simulink model "debounce_PP"  (R2017b)
settings: Solver=FixedStepDiscrete  StartTime=0.0  StopTime=10.0  RelTol=1e-3  EnableMultiTasking=on
model workspace (MAT data in the model file):
  already_pp = 1
Description:
  | Property Proving with an Assumption Block
  | 
  | This example shows how to perform a Simulink Design Verifier property proof using a
  | Proof Assumption block.
settings Model: Creator=The MathWorks, Inc.  LastModifiedBy=hbourbou
settings SolverCC: InsertRTBMode=Auto
settings DataIOCC: LimitDataPoints=on  SaveFormat=Structure
settings OptimizationCC: DefaultParameterBehavior=Inlined  ExpressionDepthLimit=2147483647  InitFltsAndDblsToZero=on  EfficientMapNaN2IntZero=off  LifeSpan=inf
settings DebuggingCC: AlgebraicLoopMsg=error  SaveWithParameterizedLinksMsg=none  UnderspecifiedInitializationDetection=Classic  MergeDetectMultiDrivingBlocksExec=none  SignalResolutionControl=TryResolveAllWithWarning  SolverPrmCheckMsg=warning  FcnCallInpInsideContextMsg=warning  StateNameClashWarn=warning  StrictBusMsg=Warning  SFUnexpectedBacktrackingDiag=warning  SFNoUnconditionalDefaultTransitionDiag=warning  SFExecutionAtInitializationDiag=none
settings HardwareCC: ProdBitPerPointer=32  ProdBitPerSizeT=32  ProdBitPerPtrDiffT=32  ProdLargestAtomicFloat=None  ProdIntDivRoundTo=Undefined  ProdEndianess=Unspecified  ProdWordSize=32  ProdHWDeviceType=32-bit Generic
settings ModelReferenceCC: PropagateSignalLabelsOutOfModel=off
settings SFSimCC: SimParseCustomCode=off
settings CodeAppCC: StateflowObjectComments=on
settings GRTTargetCC: TargetFcnLib=ansi_tfl_tmw.mat  TargetLangStandard=C89/C90 (ANSI)  GeneratePreprocessorConditionals=Disable all  CombineOutputUpdateFcns=off  GRTInterface=on
settings ConfigComp: DVMode=PropertyProving  DVMaxProcessTime=60  DVMakeOutputFilesUnique=off  DVParameters=on  DVModelCoverageObjectives=MCDC  DVMaxTestCaseSteps=500  DVTestSuiteOptimization=CombinedObjectives  DVAssertions=EnableAll  DVProofAssumptions=EnableAll  DVDetectActiveLogic=on  DVDetectFloatOverflow=off  DVProvingStrategy=FindViolation  DVModelReferenceHarness=on

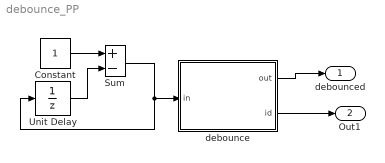
== system debounce_PP ==
  Constant : Constant  OutDataTypeStr=uint8
  Sum : Sum  Inputs=+-  OutDataTypeStr=double
  Unit Delay : UnitDelay  InitialCondition=uint8(0)  SampleTime=-1
  debounce : Stateflow chart  TreatAsAtomicUnit=on
  debounced : Outport  OutDataTypeStr=double
  Out1 : Outport  Port=2
  wires:
  Sum/1 -> Unit Delay/1, debounce/1(in)
  debounce/1(out) -> debounced/1
  debounce/2(id) -> Out1/1
  Unit Delay/1 -> Sum/2
  Constant/1 -> Sum/1

== stateflow chart debounce_PP/debounce ==
  settings: updateMethod=DISCRETE
  state To
    state To_on
      en: id = 2;
      exit: id = 0;
    state To_off
      en: id = 3;
      exit: id = 0;
  state Off
    en: out = 0 ;
    id = 1;
    exit: id = 0;
  state OnParent
    state On
      en: out = 1; id = 4;
      exit: id = 0;
  (default) -> Off
  To_on -> On [order 2] : [in==1] {out = out - 1}/{out = out + 1}
  Off -> To_on : [in==1]
  To_on -> Off [order 1] : [in==0]
  To_off -> Off [order 2] : [in==0]
  On -> To_off : [in==0]/{out =  1;}
  To_off -> On [order 1] : [in==1]
  data: in input double; out output double; id output double
